simulink model "Ball_In_The_Tube_Control"  (R2020b)
settings: Solver=VariableStepAuto  StartTime=0  StopTime=50  RelTol=1e-3
undefined symbols (not defined in the file or in its folder): InnerLoop
settings Model: Creator=Aurelien_Julien  LastModifiedBy=Aurelien_Julien

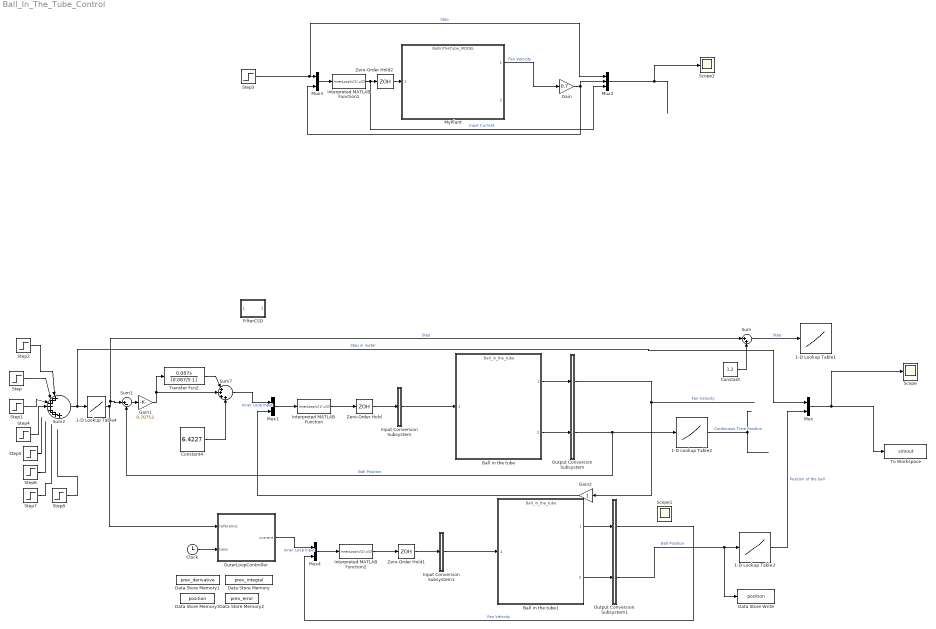
== system Ball_In_The_Tube_Control ==
  1-D Lookup Table1 : Lookup_n-D  NumberOfTableDimensions=1  BreakpointsForDimension1=[1.2 1.4 1.8 2.4 2.5 2.75 3.1 3.5 3.9 4.5 5.2 5.6 5.7 6.3 6.7 7.32]  Table=[0 15 60 97.5 117.5 125 127.5 132 135 138 142 148 152 160 167.5 180]/100  InternalRulePriority=Speed  RndMeth=Simplest  InputSameDT=on
  1-D Lookup Table2 : Lookup_n-D  NumberOfTableDimensions=1  BreakpointsForDimension1=[1.2 1.4 1.8 2.4 2.5 2.75 3.1 3.5 3.9 4.5 5.2 5.6 5.7 6.3 6.7 7.32]  Table=[0 15 60 97.5 117.5 125 127.5 132 135 138 142 148 152 160 167.5 180]/100  InternalRulePriority=Speed  RndMeth=Simplest  InputSameDT=on
  1-D Lookup Table3 : Lookup_n-D  NumberOfTableDimensions=1  BreakpointsForDimension1=[1.2 1.4 1.8 2.4 2.5 2.75 3.1 3.5 3.9 4.5 5.2 5.6 5.7 6.3 6.7 7.32]  Table=[0 15 60 97.5 117.5 125 127.5 132 135 138 142 148 152 160 167.5 180]/100  InternalRulePriority=Speed  RndMeth=Simplest  InputSameDT=on
  1-D Lookup Table4 : Lookup_n-D  NumberOfTableDimensions=1  BreakpointsForDimension1=[0 15 60 97.5 117.5 125 127.5 132 135 138 142 148 152 160 167.5 180]/100  Table=[1.2 1.4 1.8 2.4 2.5 2.75 3.1 3.5 3.9 4.5 5.2 5.6 5.7 6.3 6.7 7.32]  InternalRulePriority=Speed  RndMeth=Simplest  InputSameDT=on
  Ball in the tube : ModelReference  ModelNameDialog=Ball_in_the_tube.slxp  ModelReferenceVersion=1.11  CopyOfModelProtected=on
  Ball in the tube1 : ModelReference  ModelNameDialog=Ball_in_the_tube.slxp  ModelReferenceVersion=1.11  CopyOfModelProtected=on
  Clock : Clock
  Constant : Constant  Value=1.2
  Constant4 : Constant  Value=6.4227
  Data Store Memory : DataStoreMemory  DataStoreName=prev_integral  ReadBeforeWriteMsg=warning  WriteAfterWriteMsg=warning  WriteAfterReadMsg=warning  ShowAdditionalParam=off  OutDataTypeStr=double
  Data Store Memory1 : DataStoreMemory  DataStoreName=prev_derivative  ReadBeforeWriteMsg=warning  WriteAfterWriteMsg=warning  WriteAfterReadMsg=warning  ShowAdditionalParam=off  OutDataTypeStr=double
  Data Store Memory2 : DataStoreMemory  DataStoreName=prev_error  ReadBeforeWriteMsg=warning  WriteAfterWriteMsg=warning  WriteAfterReadMsg=warning  ShowAdditionalParam=off  OutDataTypeStr=double
  Data Store Memory3 : DataStoreMemory  DataStoreName=position  ReadBeforeWriteMsg=warning  WriteAfterWriteMsg=warning  WriteAfterReadMsg=warning  ShowAdditionalParam=off  OutDataTypeStr=double
  Data Store Write : DataStoreWrite  DataStoreName=position  SampleTime=0.01
  FilterCSD : Subsystem  Tag=FilterWizardSubSystem
      settings: ErrorFcn=dspFilterRealizedInBasicElemsAlgLoopErrFcnCallback
  Gain : Gain  Gain=0.7
  Gain1 : Gain  Gain=0.70753
  Gain2 : Gain
  Input Conversion Subsystem : Subsystem  Tag=__SLT_ICS__  Description=|
      | Signal spec.
      | and routing
      settings: AttributesFormatString=%<Description>
  Input Conversion Subsystem1 : Subsystem  Tag=__SLT_ICS__  Description=|
      | Signal spec.
      | and routing
      settings: AttributesFormatString=%<Description>
  Interpreted MATLAB Function : MATLABFcn  MATLABFcn=InnerLoop(u(1),u(2))  OutputDimensions=1
  Interpreted MATLAB Function1 : MATLABFcn  MATLABFcn=InnerLoop(u(1),u(2))  OutputDimensions=1
  Interpreted MATLAB Function2 : MATLABFcn  MATLABFcn=InnerLoop(u(1),u(2))  OutputDimensions=1
  Mux{,1,3..4} (4 alike) : Mux  Inputs=2
  Mux2 : Mux  Inputs=3
  MyPlant : ModelReference  ModelNameDialog=BallInTheTube_MODEL  SimulationMode=Normal  ModelReferenceVersion=1.2
  OuterLoopController : MATLAB Function  TreatAsAtomicUnit=on  SystemSampleTime=0.01
  Output Conversion Subsystem : Subsystem  Tag=__SLT_OCS__  Description=|
      | Signal spec.
      | and routing
      settings: AttributesFormatString=%<Description>
  Output Conversion Subsystem1 : Subsystem  Tag=__SLT_OCS__  Description=|
      | Signal spec.
      | and routing
      settings: AttributesFormatString=%<Description>
  Scope : Scope
  Scope1 : Scope
  Scope2 : Scope
  Step : Step  Time=20  After=0.1  SampleTime=0.01
  Step1 : Step  Time=30  After=0.1  SampleTime=0
  Step2 : Step  Time=10  Before=1.2  After=1.3  SampleTime=0.01
  Step3 : Step  Time=5  SampleTime=0
  Step4 : Step  Time=40  After=0.1  SampleTime=0
  Step5 : Step  Time=25  After=0.8  SampleTime=0
  Step6 : Step  Time=30  After=-0.95  SampleTime=0
  Step7 : Step  Time=35  After=0.5  SampleTime=0
  Step8 : Step  Time=40  After=-0.8  SampleTime=0
  Sum : Sum  Inputs=|++
  Sum1 : Sum  Inputs=|+-
  Sum2 : Sum  Inputs=|++++++++
  Sum7 : Sum  Inputs=|++++
  To Workspace : ToWorkspace  VariableName=simout  SaveFormat=Timeseries  SampleTime=0.01
  Transfer Fcn2 : TransferFcn  Numerator=[0.087 0]  Denominator=[0.087/5 1]
  Zero-Order Hold : ZeroOrderHold  SampleTime=0.01
  Zero-Order Hold1 : ZeroOrderHold  SampleTime=0.01
  Zero-Order Hold2 : ZeroOrderHold  SampleTime=0.01
  wires:
  Mux/1 -> Scope/1, To Workspace/1
  Interpreted MATLAB Function/1 -> Zero-Order Hold/1
  Mux1/1 -> Interpreted MATLAB Function/1
  Gain2/1 -> Mux1/2
  Sum/1 -> 1-D Lookup Table1/1  "Step"
  Ball in the tube/2 -> Output Conversion Subsystem/2(Inport_2)
  Ball in the tube/1 -> Output Conversion Subsystem/1(Inport_1)
  Input Conversion Subsystem/1(Outport_1) -> Ball in the tube/1
  Zero-Order Hold/1 -> Input Conversion Subsystem/1(Inport_1)
  Step/1 -> Sum2/2
  Step1/1 -> Sum2/3
  Step2/1 -> Sum2/1
  Output Conversion Subsystem/1(Outport_1) -> Gain2/1  "Fan Velocity"
  Step3/1 -> Mux2/1, Mux3/1  "Step"
  Mux2/1 -> Scope2/1
  MyPlant/1 -> Gain/1  "Fan Velocity"
  Mux3/1 -> Interpreted MATLAB Function1/1
  Interpreted MATLAB Function1/1 -> Mux2/3, Zero-Order Hold2/1  "Input Current"
  Gain/1 -> Mux3/2, Mux2/2
  Zero-Order Hold2/1 -> MyPlant/1
  Clock/1 -> OuterLoopController/2(time)
  Constant/1 -> Sum/2
  Sum2/1 -> Mux/1, 1-D Lookup Table4/1  "Step in meter"
  1-D Lookup Table2/1 -> ?  "Continuous Time Position"
  Step4/1 -> Sum2/4
  Step5/1 -> ?
  Step6/1 -> ?
  Step7/1 -> ?
  Step8/1 -> ?
  1-D Lookup Table4/1 -> OuterLoopController/1(reference), Sum1/1, Sum/1  "Step"
  Sum7/1 -> Mux1/1  "Inner Loop Input"
  Gain1/1 -> Transfer Fcn2/1, Sum7/2
  Transfer Fcn2/1 -> Sum7/1
  Constant4/1 -> Sum7/4
  Sum1/1 -> Gain1/1
  Output Conversion Subsystem/2(Outport_2) -> 1-D Lookup Table2/1, Sum1/2  "Ball Position"
  OuterLoopController/1(current) -> Mux4/1  "Inner Loop Input"
  Zero-Order Hold1/1 -> Input Conversion Subsystem1/1(Inport_1)
  Ball in the tube1/1 -> Output Conversion Subsystem1/1(Inport_1)
  Ball in the tube1/2 -> Output Conversion Subsystem1/2(Inport_2)
  Output Conversion Subsystem1/2(Outport_2) -> Data Store Write/1, 1-D Lookup Table3/1  "Ball Position"
  Mux4/1 -> Interpreted MATLAB Function2/1
  Interpreted MATLAB Function2/1 -> Zero-Order Hold1/1
  Input Conversion Subsystem1/1(Outport_1) -> Ball in the tube1/1
  Output Conversion Subsystem1/1(Outport_1) -> Mux4/2  "Fan Velocity"
  1-D Lookup Table3/1 -> Mux/2  "Position of the ball"

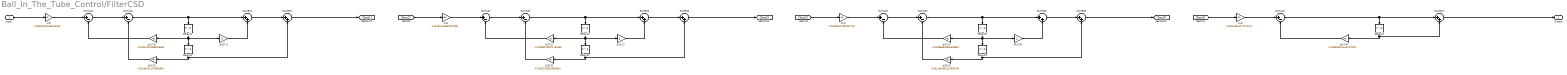
== system Ball_In_The_Tube_Control/FilterCSD ==
  Input : Inport
  Delay{11..14,21..23} (7 alike) : Delay  DelayLength=1  InitialCondition=0
  SumA{21..24,31..33} (7 alike) : Sum  Inputs=|+-  RndMeth=Nearest  SaturateOnIntegerOverflow=on  OutDataTypeStr=Inherit: Same as first input
  SumB{21..24,31..33} (7 alike) : Sum  Inputs=|++  RndMeth=Nearest  SaturateOnIntegerOverflow=on  OutDataTypeStr=Inherit: Same as first input
  a(2)(1) : Gain  Gain=-0.310670101880519356  ParamDataTypeStr=double  RndMeth=Nearest  SaturateOnIntegerOverflow=on  OutDataTypeStr=Inherit: Same as input
  a(2)(2) : Gain  Gain=-0.234801200371760499  ParamDataTypeStr=double  RndMeth=Nearest  SaturateOnIntegerOverflow=on  OutDataTypeStr=Inherit: Same as input
  a(2)(3) : Gain  Gain=-0.200856645954509805  ParamDataTypeStr=double  RndMeth=Nearest  SaturateOnIntegerOverflow=on  OutDataTypeStr=Inherit: Same as input
  a(2)(4) : Gain  Gain=-0.0955009114457573971  ParamDataTypeStr=double  RndMeth=Nearest  SaturateOnIntegerOverflow=on  OutDataTypeStr=Inherit: Same as input
  a(3)(1) : Gain  Gain=0.641364151476583655  ParamDataTypeStr=double  RndMeth=Nearest  SaturateOnIntegerOverflow=on  OutDataTypeStr=Inherit: Same as input
  a(3)(2) : Gain  Gain=0.240525788226949561  ParamDataTypeStr=double  RndMeth=Nearest  SaturateOnIntegerOverflow=on  OutDataTypeStr=Inherit: Same as input
  a(3)(3) : Gain  Gain=0.0611864362227808739  ParamDataTypeStr=double  RndMeth=Nearest  SaturateOnIntegerOverflow=on  OutDataTypeStr=Inherit: Same as input
  b(2)(1) : Gain  Gain=2  ParamDataTypeStr=double  RndMeth=Nearest  SaturateOnIntegerOverflow=on  OutDataTypeStr=Inherit: Same as input
  b(2)(2) : Gain  Gain=2  ParamDataTypeStr=double  RndMeth=Nearest  SaturateOnIntegerOverflow=on  OutDataTypeStr=Inherit: Same as input
  b(2)(3) : Gain  Gain=2  ParamDataTypeStr=double  RndMeth=Nearest  SaturateOnIntegerOverflow=on  OutDataTypeStr=Inherit: Same as input
  s(1) : Gain  Gain=0.332673512399016102  ParamDataTypeStr=double  RndMeth=Nearest  SaturateOnIntegerOverflow=on  OutDataTypeStr=Inherit: Same as input
  s(2) : Gain  Gain=0.251431146963797258  ParamDataTypeStr=double  RndMeth=Nearest  SaturateOnIntegerOverflow=on  OutDataTypeStr=Inherit: Same as input
  s(3) : Gain  Gain=0.215082447567067792  ParamDataTypeStr=double  RndMeth=Nearest  SaturateOnIntegerOverflow=on  OutDataTypeStr=Inherit: Same as input
  s(4) : Gain  Gain=0.452249544277121274  ParamDataTypeStr=double  RndMeth=Nearest  SaturateOnIntegerOverflow=on  OutDataTypeStr=Inherit: Same as input
  Output : Outport
  wires:
  Input/1 -> s(1)/1
  s(1)/1 -> SumA21/1
  SumA21/1 -> SumA31/1
  SumA31/1 -> SumB21/1, Delay11/1
  SumB21/1 -> SumB31/1
  SumB31/1 -> [Sect1]
  a(2)(1)/1 -> SumA21/2
  Delay11/1 -> a(2)(1)/1, b(2)(1)/1, Delay21/1
  b(2)(1)/1 -> SumB21/2
  a(3)(1)/1 -> SumA31/2
  Delay21/1 -> a(3)(1)/1, SumB31/2
  [Sect1] -> s(2)/1
  s(2)/1 -> SumA22/1
  SumA22/1 -> SumA32/1
  SumA32/1 -> SumB22/1, Delay12/1
  SumB22/1 -> SumB32/1
  SumB32/1 -> [Sect2]
  a(2)(2)/1 -> SumA22/2
  Delay12/1 -> a(2)(2)/1, b(2)(2)/1, Delay22/1
  b(2)(2)/1 -> SumB22/2
  a(3)(2)/1 -> SumA32/2
  Delay22/1 -> a(3)(2)/1, SumB32/2
  [Sect2] -> s(3)/1
  s(3)/1 -> SumA23/1
  SumA23/1 -> SumA33/1
  SumA33/1 -> SumB23/1, Delay13/1
  SumB23/1 -> SumB33/1
  SumB33/1 -> [Sect3]
  a(2)(3)/1 -> SumA23/2
  Delay13/1 -> a(2)(3)/1, b(2)(3)/1, Delay23/1
  b(2)(3)/1 -> SumB23/2
  a(3)(3)/1 -> SumA33/2
  Delay23/1 -> a(3)(3)/1, SumB33/2
  [Sect3] -> s(4)/1
  s(4)/1 -> SumA24/1
  SumA24/1 -> SumB24/1, Delay14/1
  SumB24/1 -> Output/1
  a(2)(4)/1 -> SumA24/2
  Delay14/1 -> a(2)(4)/1, SumB24/2

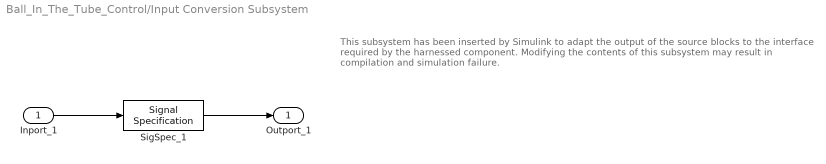
== system Ball_In_The_Tube_Control/Input Conversion Subsystem ==
  note: This subsystem has been inserted by Simulink to adapt the output of the source blocks to the interface required by the harnessed component.
      |  Modifying the contents of this subsystem may result in compilation and simulation failure.
  Inport_1 : Inport
  SigSpec_1 : SignalSpecification  OutDataTypeStr=double  Dimensions=[1]  SampleTime=[0, 1]
  Outport_1 : Outport
  wires:
  SigSpec_1/1 -> Outport_1/1
  Inport_1/1 -> SigSpec_1/1

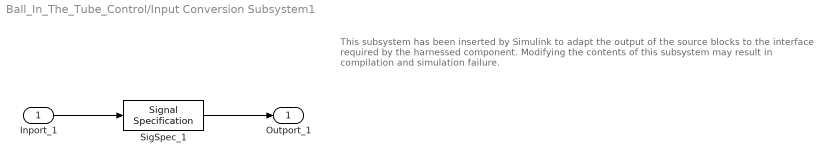
== system Ball_In_The_Tube_Control/Input Conversion Subsystem1 ==
  note: This subsystem has been inserted by Simulink to adapt the output of the source blocks to the interface required by the harnessed component.
      |  Modifying the contents of this subsystem may result in compilation and simulation failure.
  Inport_1 : Inport
  SigSpec_1 : SignalSpecification  OutDataTypeStr=double  Dimensions=[1]  SampleTime=[0, 1]
  Outport_1 : Outport
  wires:
  SigSpec_1/1 -> Outport_1/1
  Inport_1/1 -> SigSpec_1/1

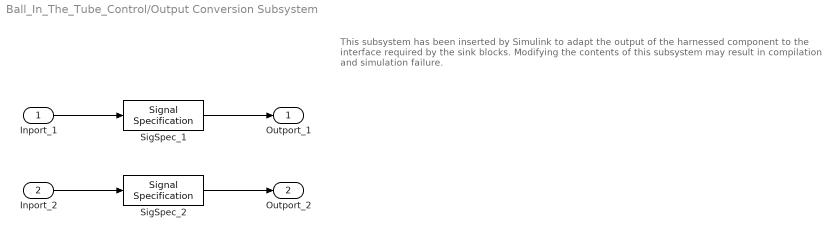
== system Ball_In_The_Tube_Control/Output Conversion Subsystem ==
  note: This subsystem has been inserted by Simulink to adapt the output of the harnessed component to the interface required by the sink blocks.
      |  Modifying the contents of this subsystem may result in compilation and simulation failure.
  Inport_1 : Inport
  Inport_2 : Inport  Port=2
  SigSpec_1 : SignalSpecification  OutDataTypeStr=double  Dimensions=[1]
  SigSpec_2 : SignalSpecification  OutDataTypeStr=double  Dimensions=[1]
  Outport_1 : Outport
  Outport_2 : Outport  Port=2
  wires:
  Inport_1/1 -> SigSpec_1/1
  SigSpec_1/1 -> Outport_1/1
  Inport_2/1 -> SigSpec_2/1
  SigSpec_2/1 -> Outport_2/1

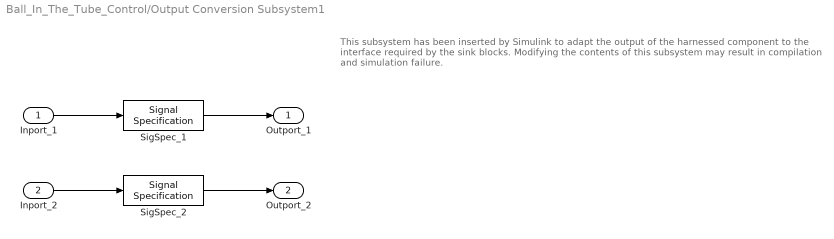
== system Ball_In_The_Tube_Control/Output Conversion Subsystem1 ==
  note: This subsystem has been inserted by Simulink to adapt the output of the harnessed component to the interface required by the sink blocks.
      |  Modifying the contents of this subsystem may result in compilation and simulation failure.
  Inport_1 : Inport
  Inport_2 : Inport  Port=2
  SigSpec_1 : SignalSpecification  OutDataTypeStr=double  Dimensions=[1]
  SigSpec_2 : SignalSpecification  OutDataTypeStr=double  Dimensions=[1]
  Outport_1 : Outport
  Outport_2 : Outport  Port=2
  wires:
  Inport_1/1 -> SigSpec_1/1
  SigSpec_1/1 -> Outport_1/1
  Inport_2/1 -> SigSpec_2/1
  SigSpec_2/1 -> Outport_2/1

== matlab function Ball_In_The_Tube_Control/OuterLoopController ==
  data: reference input; current output; time input; prev_integral data_store_memory; prev_derivative data_store_memory; prev_error data_store_memory; position data_store_memory
function current = OuterLoopController(reference,time)
global prev_integral;
global prev_derivative;
global prev_error;
global position;

if(time == 0)
   prev_error = 0;
   prev_integral = 0;
   prev_derivative = 0;
end

Ki = 0.1;
Ts = 0.01;
Kd = 0.1;

if (position < 2.5)
    Kp = 5.0766;
else
    Kp = 0.70753;
end

error = reference - position;
integral = 0;
derivative = prev_derivative*0.5536+3.884*error-3.884*prev_error;
current = Kp*error + Kp*integral + Kp*derivative;

prev_integral = integral;
prev_derivative = derivative;
prev_error = error;

current = current + 6.4227;

if(abs(current)>10)
    current = 10*sign(current);
end

end
